simulink model "simul4"  (Simulink 8.8)
settings: Solver=VariableStepAuto  StartTime=0.0  StopTime=50  RelTol=1e-3
settings Model: Creator=mebuffet  LastModifiedBy=mebuffet
settings DataIOCC: LimitDataPoints=off  SaveFormat=Dataset  SignalLoggingSaveFormat=Dataset
settings OptimizationCC: LifeSpan=auto
settings DebuggingCC: UnderspecifiedInitializationDetection=Simplified  MergeDetectMultiDrivingBlocksExec=error  FcnCallInpInsideContextMsg=error  StateNameClashWarn=none  SFUnexpectedBacktrackingDiag=error  SFNoUnconditionalDefaultTransitionDiag=error  SFExecutionAtInitializationDiag=warning
settings HardwareCC: ProdBitPerPointer=64  ProdBitPerSizeT=64  ProdBitPerPtrDiffT=64  ProdLargestAtomicFloat=Float  ProdIntDivRoundTo=Zero  ProdEndianess=LittleEndian  ProdWordSize=64  ProdHWDeviceType=Intel->x86-64 (Windows64)
settings ModelReferenceCC: PropagateSignalLabelsOutOfModel=on
settings GRTTargetCC: TargetLangStandard=C99 (ISO)  GeneratePreprocessorConditionals=Use local settings  CombineOutputUpdateFcns=on  GRTInterface=off
settings ConfigComp: CovMetricSettings=dwe  CovHtmlReporting=off  CovSaveCumulativeToWorkspaceVar=off  CovSaveSingleToWorkspaceVar=off  CovExternalEMLEnable=on

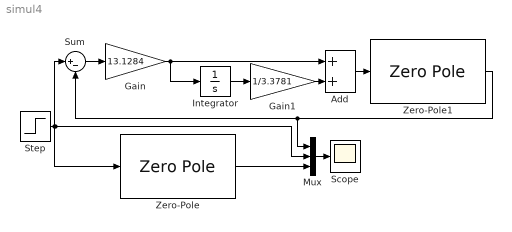
== system simul4 ==
  Add : Sum
  Gain : Gain  Gain=13.1284
  Gain1 : Gain  Gain=1/3.3781
  Integrator : Integrator
  Mux : Mux  Inputs=3
  Scope : Scope
  Step : Step  SampleTime=0
  Sum : Sum  Inputs=|+-
  Zero-Pole : ZeroPole  Zeros=[]  Poles=[-0.9 -0.9 -0.9]  Gain=[0.2]
  Zero-Pole1 : ZeroPole  Zeros=[]  Poles=[-0.9 -0.9 -0.9]  Gain=[0.2]
  wires:
  Mux/1 -> Scope/1
  Step/1 -> Zero-Pole/1, Sum/1, Mux/2
  Zero-Pole/1 -> Mux/3
  Zero-Pole1/1 -> Sum/2, Mux/1
  Sum/1 -> Gain/1
  Gain/1 -> Integrator/1, Add/1
  Add/1 -> Zero-Pole1/1
  Integrator/1 -> Gain1/1
  Gain1/1 -> Add/2
